simulink model "model_regulator2"  (R2024a)
settings: Solver=FixedStepAuto  StartTime=0.0  StopTime=10.0  FixedStep=0.001  RelTol=1e-3
undefined symbols (not defined in the file): k0, k1, T
settings Model: Creator=main  LastModifiedBy=main

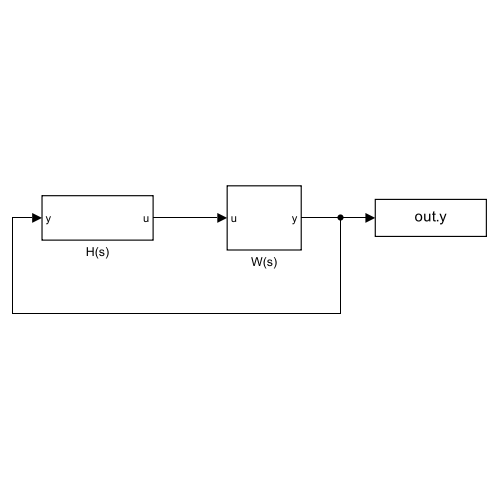
[thumbnail: Simulink's stored preview of the top-level diagram]
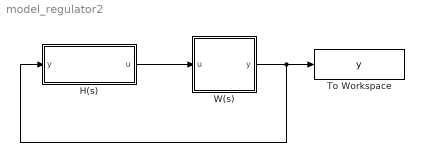
== system model_regulator2 ==
  H(s) : Subsystem
  To Workspace : ToWorkspace  VariableName=y  SaveFormat=Timeseries  SampleTime=-1
  W(s) : Subsystem
  wires:
  W(s)/1(y) -> H(s)/1(y), To Workspace/1
  H(s)/1(u) -> W(s)/1(u)

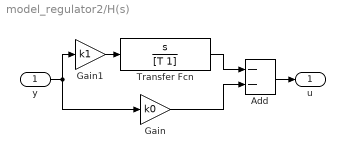
== system model_regulator2/H(s) ==
  y : Inport
  Add : Sum  Inputs=--
  Gain : Gain  Gain=k0
  Gain1 : Gain  Gain=k1
  Transfer Fcn : TransferFcn  Numerator=[1 0]  Denominator=[T 1]
  u : Outport
  wires:
  y/1 -> Gain/1, Gain1/1
  Add/1 -> u/1
  Gain/1 -> Add/2
  Gain1/1 -> Transfer Fcn/1
  Transfer Fcn/1 -> Add/1

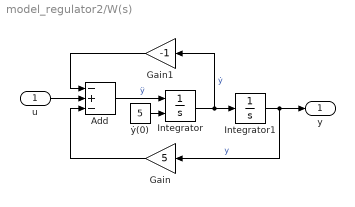
== system model_regulator2/W(s) ==
  u : Inport
  Add : Sum  Inputs=-+-
  Gain : Gain  Gain=5
  Gain1 : Gain  Gain=-1
  Integrator : Integrator  InitialConditionSource=external  InitialCondition=5
  Integrator1 : Integrator
  ẏ(0) : Constant  Value=5
  y : Outport
  wires:
  Integrator1/1 -> y/1, Gain/1  "y"
  Add/1 -> Integrator/1  "ÿ"
  Gain/1 -> Add/3
  Integrator/1 -> Gain1/1, Integrator1/1  "ẏ"
  Gain1/1 -> Add/1
  ẏ(0)/1 -> Integrator/2
  u/1 -> Add/2
